simulink model "final_LIithium_inductionmotor_powered_vehicle"  (R2020a)
settings: Solver=VariableStepAuto  StartTime=0  StopTime=240  RelTol=1e-3
libraries: autolibshared x4, autolibdatasheetbattery x1, autolibim x1, simulink x1, autolibmotorctrlr x1, autolibinverter x1, autolibshareddiff x1, autolibsharedcoupling x1
(part 3 of 3)

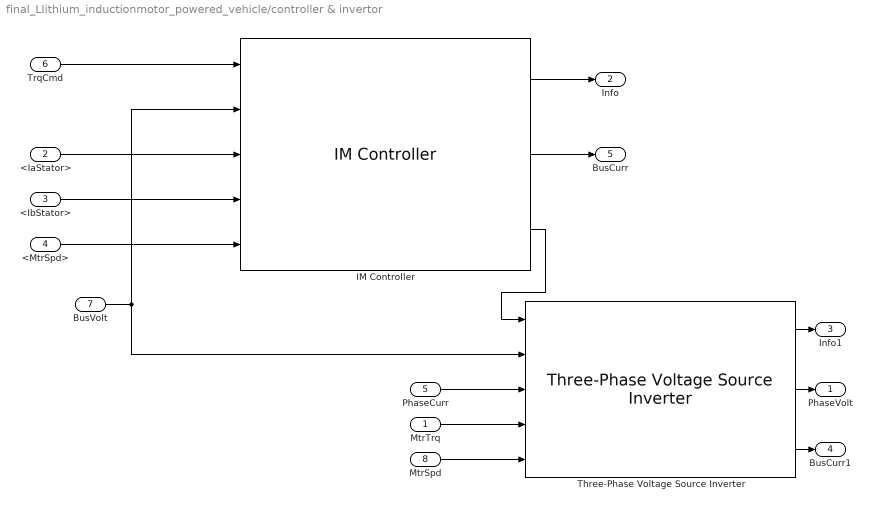
== system final_LIithium_inductionmotor_powered_vehicle/controller & invertor ==
  MtrTrq : Inport
  <IaStator> : Inport  Port=2
  <IbStator> : Inport  Port=3
  <MtrSpd> : Inport  Port=4
  PhaseCurr : Inport  Port=5
  TrqCmd : Inport  Port=6
  BusVolt : Inport  Port=7
  MtrSpd : Inport  Port=8
  IM Controller : autolibmotorctrlr/IM Controller  control_type=Torque Control  Rs=1.77  Lls=0.0139  Rr=1.34  Llr=0.0121  Lm=0.3687  PolePairs=4  Mechanical=[0.025, 0, 0]  Frate=60  Vrate=460  Srate=0.0172  Isd_0=3.1004  Isq_0=5.7131  Tem=12.6467  EV_current=200  Tst=5e-5  Kp=32.1894  Ki=2224.2476  EV_motion=[20, 4, 0.8]  EV_sf=200  ba=3.8804  Ksa=97.5161  Kisa=395.338  Ksf=373.4603  Jcomp=0.025  Fv=0  Fs=0  param_loss=Single efficiency measurement  eff=98  w_loss_bp=[0 200 400 600 800 1000]  T_loss_bp=[0 25 50 75 100]  losses_table=[100 100 100 100 100;100 150 200 250 300;100 200 300 400 500;100 250 400 550 700;100 300 500 700 900;100 350 600 850 1100]  w_eff_bp=[200 400 600 800 1000]  T_eff_bp=[25 50 75 100]  efficiency_table=[96.2 98.1 98.7 99;98.1 99 99.4 99.5;98.7 99.4 99.6 99.7;99 99.5 99.7 99.8;99.2 99.6 99.7 99.8]  x_w_bp=0  x_T_bp=0  x_losses_mat=0  Tsm=5e-4
      settings: SourceProductName=Powertrain Blockset
  Three-Phase Voltage Source Inverter : autolibinverter/Three-Phase Voltage Source Inverter  InvrtrTmpInpEnbl=off  enable_hdl=off  model_type=Commanded phase voltage  fs=10000  w_eff_bp=[-1000 -500 0 500 1000]  n1=128  T_eff_bp=[-200 -100 0 100 200]  Temp_eff_bp=[213.15 293.15 373.15]  n2=128  ploss_table=[1 0.999 0.989 0.997 0.996;0.995 0.994 0.993 0.992 0.991;0.990 0.989 0.988 0.987 0.986;0.985 0.984 0.983 0.982 0.981;0.980 0.979 0.978 0.977 0.976]  ploss_table_3d=cat(3,0.95*[1 0.999 0.989 0.997 0.996;0.995 0.994 0.993 0.992 0.991;0.990 0.989 0.988 0.987 0.986;0.985 0.984 0.983 0.982 0.981;0.980 0.979 0.978 0.977 0.976],[1 0.999 0.989 0.997 0.996;0.995 0.994 0.993 0.992 0.991;0.990 0.989 0.988 0.987 0.986;0.985 0.984 0.983 0.982 0.981;0.980 0.979 0.978 0.977 0.976],0.92*[1 0.999 0.989 0.997 0.996;0.995 0.994 0.993 0.992 0.991;0.990 0.989 0.988 0.987 0.986;0.985 0.984 0.983 0.982 0.981;0.980 0.979 0.978 0.977 0.976])  preExtrapFlag=off  u1max=1000  u1min=-1000  u2max=200  u2min=-200  intPrec=23  RefBlkName='autolibmappedmotor/Mapped Motor'  CalLossMapData={}  CalLossWithTempMapData={}
      settings: SourceProductBaseCode=PW,MT,VE,VP
  PhaseVolt : Outport
  Info : Outport  Port=2
  Info1 : Outport  Port=3
  BusCurr1 : Outport  Port=4
  BusCurr : Outport  Port=5
  wires:
  BusVolt/1 -> IM Controller/2, Three-Phase Voltage Source Inverter/2
  IM Controller/3 -> Three-Phase Voltage Source Inverter/1
  PhaseCurr/1 -> Three-Phase Voltage Source Inverter/3
  TrqCmd/1 -> IM Controller/1
  MtrSpd/1 -> Three-Phase Voltage Source Inverter/5
  MtrTrq/1 -> Three-Phase Voltage Source Inverter/4
  <MtrSpd>/1 -> IM Controller/5
  <IaStator>/1 -> IM Controller/3
  <IbStator>/1 -> IM Controller/4
  IM Controller/2 -> BusCurr/1
  Three-Phase Voltage Source Inverter/2 -> PhaseVolt/1
  Three-Phase Voltage Source Inverter/3 -> BusCurr1/1
  Three-Phase Voltage Source Inverter/1 -> Info1/1
  IM Controller/1 -> Info/1

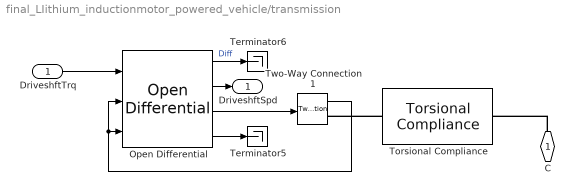
== system final_LIithium_inductionmotor_powered_vehicle/transmission ==
  DriveshftTrq : Inport
  Open Differential : autolibshareddiff/Open Differential  DiffEffModelPopup=Constant  InterpMethod=Linear point-slope  extTamb=off  shaftSwitchMask=To the left of center-line  Ndiff=9.34  Jd=.025  bd=1e-3  Jw1=.01  bw1=1e-3  Jw2=.01  bw2=1e-3  omegaw1o=0  omegaw2o=0  eta=1  eta_tbl=reshape([0.64 0.76 0.8 0.81 0.83 0.84 0.84 0.56 0.73 0.78 0.8 0.83 0.84 0.84 0.54 0.71 0.77 0.8 0.82 0.84 0.84 0.53 0.71 0.77 0.8 0.83 0.84 0.84 0.51 0.71 0.77 0.8 0.83 0.84 0.85 0.52 0.7 0.77 0.8 0.83 0.84 0.85 0.51 0.71 0.76 0.79 0.83 0.84 0.85 0.5 0.69 0.76 0.79 0.82 0.84 0.85 0.45 0.68 0.75 0.78 0.82 0.84 0.85 0.43 0.67 0.74 0.78 0.81 0.83 0.84 0.38 0.63 0.71 0.75 0.8 0.82 0.83 0.81 0.86 0.88 0.89 0.89 0.89 0.9 0.77 0.85 0.87 0.88 0.89 0.9 0.9 0.72 0.82 0.86 0.87 0.88 0.89 0.9 0.68 0.8 0.84 0.86 0.88 0.89 0.89 0.67 0.8 0.84 0.86 0.88 0.89 0.9 0.67 0.8 0.84 0.86 0.88 0.89 0.9 0.65 0.8 0.84 0.86 0.88 0.89 0.9 0.64 0.79 0.83 0.86 0.88 0.89 0.9 0.63 0.78 0.83 0.86 0.88 0.89 0.9 0.59 0.76 0.82 0.85 0.87 0.89 0.9 0.53 0.73 0.8 0.83 0.86 0.88 0.89], 7, 11, 2)  Trq_bpts=[25, 50, 75, 100, 150, 200, 250]  omega_bpts=[52.4 78.5 105 131 157 183 209 262 314 419 524]  Temp_bpts=[290 358]  Tamb=297.15  maxAbsSpd=5e3  aMode=aMode
      settings: SourceProductBaseCode=PW
  Terminator5 : Terminator
  Terminator6 : Terminator
  Torsional Compliance : autolibsharedcoupling/Torsional Compliance  port_config=Two-way connection  extInfo=off  k=1e4  b=1e2  theta_o=0  domega_o=0  omega_c=3000  blkID=0  aMode=1
      settings: SourceProductBaseCode=PW,MT,VE,VP
  Two-Way Connection1 : TwoWayConnection
  C : PMIOPort  Side=Right
  DriveshftSpd : Outport
  wires:
  DriveshftTrq/1 -> Open Differential/1
  Open Differential/3 -> Two-Way Connection1/1
  Open Differential/1 -> Terminator6/1  "Diff"
  Two-Way Connection1/1 -> Open Differential/2, Open Differential/3
  Open Differential/4 -> Terminator5/1
  Open Differential/2 -> DriveshftSpd/1
  connections:
  Torsional Compliance/LConn1 -- Two-Way Connection1/RConn1
  C/RConn1 -- Torsional Compliance/RConn1
